simulink model "Shanthan_Heeirthan_EE469S3D_R45 (1)"  (R2023a)
settings: Solver=FixedStepDiscrete  StartTime=0.0  StopTime=120  FixedStep=dt0  RelTol=1e-3  EnableMultiTasking=on
PostLoadFcn:
  | %Set the size for the model
  | set_param(gcs,'Location',[10 10 1270 970])
  | %Set the zoom factor for the model
  | set_param(gcs,'ZoomFactor','100')
InitFcn:
  | tic
  | % Students Add call to their M-file HERE
  | Shanthan_Heeirthan_EE460_Final
  | INIT_S3D_01
StartFcn:
  | tend0=toc;
  | tic;
StopFcn:
  | tend=toc;
  | disp(['Simulation time = ' num2str(tout(end)) ' sec'])
  | disp(['Real time = ' num2str(tend) ' sec'])
  | title('DONE')
  | SCORE=round((max(0,120-tout(end)-tend0))*4+10*(40-FuelBurned)+sum(100*double(PDONE)-100*double(PDONE<.5)));
  | PlotS3D(PlotInput);
  | text(15,22,['S: ' num2str(SCORE)]);
values from neighbouring files (symbols this model uses):
  A = [0 1 0 0 0 0 ... (first row only)    [Shanthan_Heeirthan_EE460_Final (1).m]
  B = [0 0 0 ... (first row only)    [Shanthan_Heeirthan_EE460_Final (1).m]
  bm = [1 1 -1 -1 0 0 0 0; 0 0 0 0 -1 1 1 -1; -1 1 -1 1 3 -3 3 -3]    [Shanthan_Heeirthan_EE460_Final (1).m]
  C = [1 0 0 0 0 0 ... (first row only)    [Shanthan_Heeirthan_EE460_Final (1).m]
  D = [0 0 0 ... (first row only)    [Shanthan_Heeirthan_EE460_Final (1).m]
  Denchptheta = TFchptheta.Den{1}    [Shanthan_Heeirthan_EE460_Final (1).m]
  Denchpxy = TFchpxy.Den{1}    [Shanthan_Heeirthan_EE460_Final (1).m]
  Denclptheta = TFclptheta.Den{1}    [Shanthan_Heeirthan_EE460_Final (1).m]
  Denclpxy = TFclpxy.Den{1}    [Shanthan_Heeirthan_EE460_Final (1).m]
  Denlp = TFlp.Den{1}    [Shanthan_Heeirthan_EE460_Final (1).m]
  Kd = 2.1+0    (= 2.1)    [Shanthan_Heeirthan_EE460_Final (1).m]
  Ki = 0.0001    [Shanthan_Heeirthan_EE460_Final (1).m]
  Kp = 1.1+0.2    (= 1.3)    [Shanthan_Heeirthan_EE460_Final (1).m]
  L = place(A',C',ep)'    [Shanthan_Heeirthan_EE460_Final (1).m]
  Numchptheta = TFchptheta.Num{1}    [Shanthan_Heeirthan_EE460_Final (1).m]
  Numchpxy = TFchpxy.Num{1}    [Shanthan_Heeirthan_EE460_Final (1).m]
  Numclptheta = TFclptheta.Num{1}    [Shanthan_Heeirthan_EE460_Final (1).m]
  Numclpxy = TFclpxy.Num{1}    [Shanthan_Heeirthan_EE460_Final (1).m]
  Numlp = TFlp.Num{1}    [Shanthan_Heeirthan_EE460_Final (1).m]
  Pnewdata = [LVL.P1 LVL.P2 LVL.P3 LVL.P4]    [Shanthan_Heeirthan_EE460_Final (1).m]
  Sconfig = 1    [Shanthan_Heeirthan_EE460_Final (1).m]
  TFP1 = 2    [Shanthan_Heeirthan_EE460_Final (1).m]
  TFP1z = 1    [Shanthan_Heeirthan_EE460_Final (1).m]
  TFP2 = 2    [Shanthan_Heeirthan_EE460_Final (1).m]
  TFP2z = 1    [Shanthan_Heeirthan_EE460_Final (1).m]
  TFP3 = 2    [Shanthan_Heeirthan_EE460_Final (1).m]
  TFP3z = 1    [Shanthan_Heeirthan_EE460_Final (1).m]
  TFP4 = 2    [Shanthan_Heeirthan_EE460_Final (1).m]
  TFP4z = 1    [Shanthan_Heeirthan_EE460_Final (1).m]
  wcf = 2    [Shanthan_Heeirthan_EE460_Final (1).m]
  wcft = 10    [Shanthan_Heeirthan_EE460_Final (1).m]
undefined symbols (not defined in the file or in its folder): d2r, DiscIntNeverNeededParam, dt, dt0, fr, HM_S, HM_U, J, Jbase, JC0, L13, L24, LVL, M, M1, M2, M3, M4, mdti, Pdata, PTvec, r2d, SLIM, SQ, SSF, TOLdata, ULIM
libraries: simulink x85, aerolibanimutils x1, matrix_library x1
(part 1 of 7)
settings Model: Creator=bordignk  LastModifiedBy=shanthah
settings SolverCC: AlgebraicLoopSolver=TrustRegion  AutoInsertRateTranBlk=on
settings DataIOCC: LimitDataPoints=on  SaveFormat=Array  ReturnWorkspaceOutputs=off
settings OptimizationCC: LifeSpan=inf
settings DebuggingCC: CheckSSInitialOutputMsg=off  UnderspecifiedInitializationDetection=Classic  MergeDetectMultiDrivingBlocksExec=none  ParameterPrecisionLossMsg=none  AllowSymbolicDim=off  StateNameClashWarn=warning  SFUnexpectedBacktrackingDiag=warning  SFNoUnconditionalDefaultTransitionDiag=warning  SFExecutionAtInitializationDiag=none  ArithmeticOperatorsInVariantConditions=warning
settings HardwareCC: ProdBitPerPointer=32  ProdBitPerSizeT=32  ProdBitPerPtrDiffT=32  ProdLargestAtomicFloat=None  ProdIntDivRoundTo=Undefined  ProdEndianess=Unspecified  ProdWordSize=32  ProdHWDeviceType=32-bit Generic
settings ModelReferenceCC: EnableRefExpFcnMdlSchedulingChecks=on  PropagateSignalLabelsOutOfModel=off
settings SFSimCC: SimUseLocalCustomCode=off  CustomCodeUndefinedFunction=UseInterfaceOnly
settings RTWCC: RTWUseLocalCustomCode=off  DLArmComputeVersion=19.05
settings CodeAppCC: StateflowObjectComments=on
settings GRTTargetCC: TargetLangStandard=C89/C90 (ANSI)
settings ConfigComp: CovMetricSettings=dw  CovSaveCumulativeToWorkspaceVar=on  CovSaveSingleToWorkspaceVar=on  CovExternalEMLEnable=off

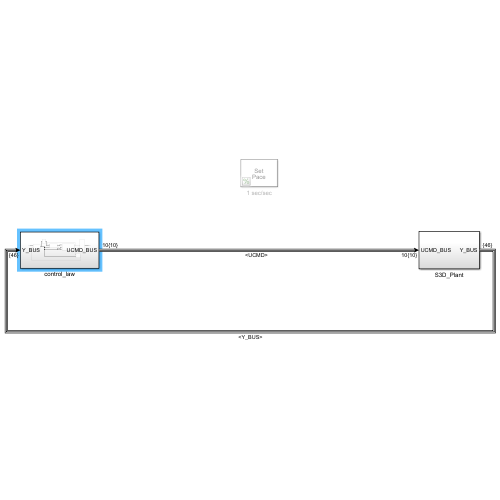
[thumbnail: Simulink's stored preview of the top-level diagram]
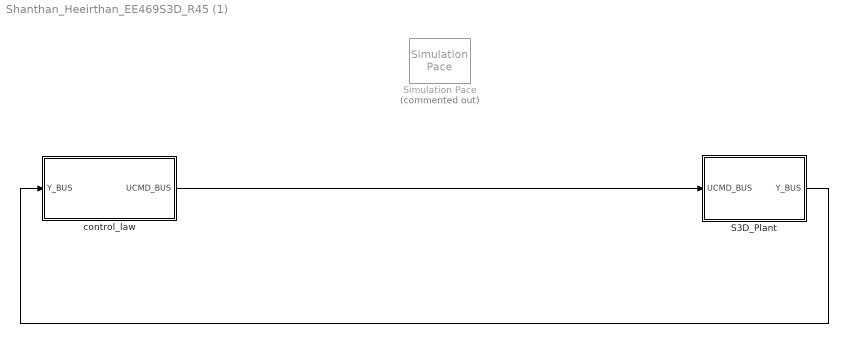
== system Shanthan_Heeirthan_EE469S3D_R45 (1) ==
  S3D_Plant : Subsystem
  Simulation Pace : aerolibanimutils/Simulation Pace  Commented=on  SimulationPace=1  SleepMode=MATLAB Thread  OutputPaceError=off  SampleTime=-1
      settings: AttributesFormatString=%<SimulationPace> sec/sec
  control_law : Subsystem
  wires:
  control_law/1(UCMD_BUS) -> S3D_Plant/1(UCMD_BUS)
  S3D_Plant/1(Y_BUS) -> control_law/1(Y_BUS)

== system Shanthan_Heeirthan_EE469S3D_R45 (1)/S3D_Plant ==
  UCMD_BUS : Inport
  Comm : Subsystem
  GetAccel : Subsystem
  Integrate : Subsystem
  MassProperties : Subsystem
  OutputDataProcessing : Subsystem
  Sensors : Subsystem
  ThrusterValues : Subsystem
  Y_BUS : Outport
  wires:
  Integrate/1(XCentroid) -> OutputDataProcessing/4(x), Comm/1(X), Sensors/1(X), GetAccel/3(X)
  MassProperties/1(MP) -> OutputDataProcessing/1(MP), Integrate/1(MP), GetAccel/1(MP), ThrusterValues/1(MP)
  OutputDataProcessing/1(Y_BUS) -> Y_BUS/1
  Comm/1(COMM) -> OutputDataProcessing/3(COMM)
  Sensors/1(Sensors) -> OutputDataProcessing/2(Sensors)
  ThrusterValues/1(U) -> MassProperties/1(U), OutputDataProcessing/5(U), GetAccel/2(U)
  GetAccel/1(ACCEL) -> Integrate/2(ACCEL)
  UCMD_BUS/1 -> ThrusterValues/2(UCMD_BUS)

== system Shanthan_Heeirthan_EE469S3D_R45 (1)/control_law ==
  Y_BUS : Inport
  Bus Selector : BusSelector  OutputSignals=Ufail  OutputAsBus=on
  CMD : Subsystem
  InputDataConditioning : Subsystem
  Observer : Subsystem
  OutputDataConditioning : Subsystem
  Regulator : Subsystem
  thrustercmd : Subsystem
  UCMD_BUS : Outport
  wires:
  Y_BUS/1 -> InputDataConditioning/1(Y_BUS)
  OutputDataConditioning/1(UCMD_BUS) -> UCMD_BUS/1
  thrustercmd/1(U_lim) -> Regulator/1(U_lim), OutputDataConditioning/1(U_lim)
  InputDataConditioning/1(Y_IN) -> Observer/2(Y_IN), Bus Selector/1, thrustercmd/3(Y_IN), Regulator/3(Y_IN), CMD/1(Y_IN)
  Regulator/1(Up) -> thrustercmd/1(Up)
  CMD/1(CMD) -> Regulator/2(CMD)
  thrustercmd/2(CAout) -> Observer/1(CAout)
  Observer/1(xhat) -> InputDataConditioning/2(x_hat)
  Bus Selector/1 -> thrustercmd/2(Ufail)  "Ufail"

== system Shanthan_Heeirthan_EE469S3D_R45 (1)/S3D_Plant/Comm ==
  X : Inport
  Bus Creator : BusCreator  Inputs=8
  Bus Selector : BusSelector  OutputSignals=P1Done,P2Done,P3Done,P4Done  OutputAsBus=on
  Bus Selector1 : BusSelector  OutputSignals=P1Done,P2Done,P3Done,P4Done  OutputAsBus=on
  Compare To Constant : simulink/Logic and Bit Operations/Compare To Constant  relop=>=  const=4  OutDataTypeStr=boolean
  Data Type Conversion : DataTypeConversion  OutDataTypeStr=uint8  SaturateOnIntegerOverflow=off  RndMeth=Floor
  P1 : Subsystem  mask{Pdx=1}
      mask prompts: Pdx "Data Point (1-4)"
  P2 : Subsystem  mask{Pdx=2}
      mask prompts: Pdx "Data Point (1-4)"
  P3 : Subsystem  mask{Pdx=3}
      mask prompts: Pdx "Data Point (1-4)"
  P4 : Subsystem  mask{Pdx=4}
      mask prompts: Pdx "Data Point (1-4)"
  Stop Simulation : Stop
  Sum of Elements : Sum  Inputs=+
  To Workspace : ToWorkspace  VariableName=PDONE  SampleTime=dt0
      settings: MaxDataPoints=1
  COMM : Outport
  wires:
  Compare To Constant/1 -> Stop Simulation/1
  Sum of Elements/1 -> Compare To Constant/1
  Data Type Conversion/1 -> Sum of Elements/1
  Bus Selector1/1 -> Data Type Conversion/1
  Bus Selector/1 -> To Workspace/1  "PDONE"
  Bus Creator/1 -> COMM/1, Bus Selector/1, Bus Selector1/1  "COMM"
  P4/1(COMM_OK) -> Bus Creator/7  "P4OK"
  P4/2(COMM_DONE) -> Bus Creator/8  "P4Done"
  P3/1(COMM_OK) -> Bus Creator/5  "P3OK"
  P3/2(COMM_DONE) -> Bus Creator/6  "P3Done"
  P2/1(COMM_OK) -> Bus Creator/3  "P2OK"
  P2/2(COMM_DONE) -> Bus Creator/4  "P2Done"
  P1/2(COMM_DONE) -> Bus Creator/2  "P1Done"
  P1/1(COMM_OK) -> Bus Creator/1  "P1OK"
  X/1 -> P3/1(X), P4/1(X), P2/1(X), P1/1(X)

== system Shanthan_Heeirthan_EE469S3D_R45 (1)/S3D_Plant/GetAccel ==
  MP : Inport
  U : Inport  Port=2
  X : Inport  Port=3
  Bus Creator : BusCreator  Inputs=3
  GetFxb : Subsystem
  GetFyb : Subsystem
  GetMz : Subsystem
  InertialAccel : Subsystem
  ACCEL : Outport
  wires:
  InertialAccel/1(ACCEL) -> ACCEL/1
  Bus Creator/1 -> InertialAccel/1(FM)  "FM"
  MP/1 -> GetMz/2(MP), InertialAccel/2(MP)
  X/1 -> InertialAccel/3(X)
  U/1 -> GetFxb/1(U), GetFyb/1(U), GetMz/1(U)
  GetFxb/1(Fxb) -> Bus Creator/1
  GetFyb/1(Fyb) -> Bus Creator/2
  GetMz/1(Mzb) -> Bus Creator/3

== system Shanthan_Heeirthan_EE469S3D_R45 (1)/S3D_Plant/Integrate ==
  MP : Inport
  ACCEL : Inport  Port=2
  ABM_INT1 : Subsystem
  Bus Creator : BusCreator  Inputs=9
  Bus Selector2 : BusSelector  OutputSignals=xddt_mps2,yddt_mps2,thtddt_rps2
  Bus to Vector1 : BusToVector
  CentroidData : Subsystem
  Demux : Demux  Outputs=6
  Mux : Mux  Inputs=2
  Selector : Selector  InputPortWidth=6  IndexOptions=Index vector (dialog)  Indices=[4 5 6]  OutputSizes=1
  XCentroid : Outport
  wires:
  CentroidData/1(XCentroid) -> XCentroid/1
  MP/1 -> CentroidData/1(MP)
  Bus Selector2/3 -> Bus Creator/9  "<thtddt_rps2>"
  Bus Selector2/1 -> Bus Creator/7  "<xddt_mps2>"
  Bus Selector2/2 -> Bus Creator/8  "<yddt_mps2>"
  Bus to Vector1/1 -> Mux/2
  Bus Creator/1 -> CentroidData/2(XCG)  "XCG"
  Selector/1 -> Mux/1
  ACCEL/1 -> Bus to Vector1/1, Bus Selector2/1
  Demux/4 -> Bus Creator/4  "xdt_mps"
  Demux/6 -> Bus Creator/6  "thtdt_rps"
  Demux/5 -> Bus Creator/5  "ydt_mps"
  Demux/2 -> Bus Creator/2  "y_m"
  Demux/1 -> Bus Creator/1  "x_m"
  Demux/3 -> Bus Creator/3  "tht_rad"
  Mux/1 -> ABM_INT1/1(DX)  "DX"
  ABM_INT1/1(X) -> Selector/1, Demux/1

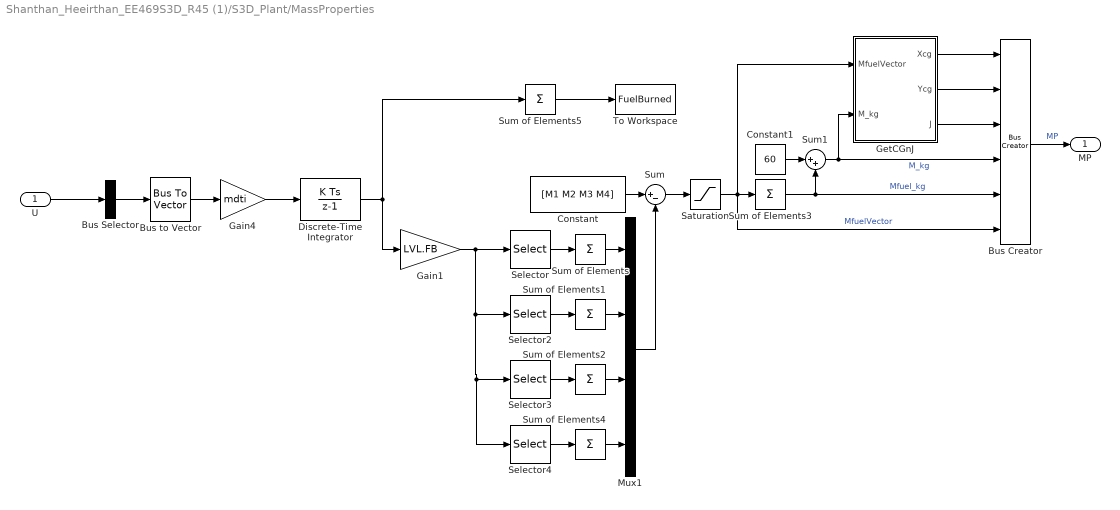
== system Shanthan_Heeirthan_EE469S3D_R45 (1)/S3D_Plant/MassProperties ==
  U : Inport
  Bus Creator : BusCreator  Inputs=6
  Bus Selector : BusSelector  OutputSignals=U1,U2,U3,U4,U5,U6,U7,U8  OutputAsBus=on
  Bus to Vector : BusToVector
  Constant : Constant  Value=[M1 M2 M3 M4]  SampleTime=dt0
  Constant1 : Constant  Value=60  SampleTime=dt0
  Discrete-Time Integrator : DiscreteIntegrator  SampleTime=dt0  UpperSaturationLimit=10  LowerSaturationLimit=0  ICPrevOutput=DiscIntNeverNeededParam  ICPrevScaledInput=DiscIntNeverNeededParam
  Gain1 : Gain  Gain=LVL.FB
  Gain4 : Gain  Gain=mdti
  GetCGnJ : Subsystem
  Mux1 : Mux
  Saturation : Saturate  UpperLimit=10  LowerLimit=0
  Selector : Selector  InputPortWidth=8  IndexOptions=Index vector (dialog)  Indices=[1 5]  OutputSizes=1
  Selector2 : Selector  InputPortWidth=8  IndexOptions=Index vector (dialog)  Indices=[2 6]  OutputSizes=1
  Selector3 : Selector  InputPortWidth=8  IndexOptions=Index vector (dialog)  Indices=[3 7]  OutputSizes=1
  Selector4 : Selector  InputPortWidth=8  IndexOptions=Index vector (dialog)  Indices=[4 8]  OutputSizes=1
  Sum : Sum  Inputs=|+-
  Sum of Elements{,1..5} (6 alike) : Sum  Inputs=+
  Sum1 : Sum  Inputs=|++
  To Workspace : ToWorkspace  VariableName=FuelBurned  SampleTime=dt0
      settings: MaxDataPoints=1
  MP : Outport
  wires:
  Gain1/1 -> Selector/1, Selector2/1, Selector3/1, Selector4/1
  Bus Creator/1 -> MP/1  "MP"
  GetCGnJ/3(J) -> Bus Creator/3
  GetCGnJ/2(Ycg) -> Bus Creator/2
  GetCGnJ/1(Xcg) -> Bus Creator/1
  Sum1/1 -> GetCGnJ/2(M_kg), Bus Creator/4  "M_kg"
  Sum of Elements3/1 -> Bus Creator/5, Sum1/2  "Mfuel_kg"
  Constant1/1 -> Sum1/1
  Saturation/1 -> Sum of Elements3/1, GetCGnJ/1(MfuelVector), Bus Creator/6  "MfuelVector"
  Sum/1 -> Saturation/1
  Constant/1 -> Sum/1
  Bus Selector/1 -> Bus to Vector/1
  U/1 -> Bus Selector/1
  Sum of Elements/1 -> Mux1/1
  Selector4/1 -> Sum of Elements4/1
  Selector3/1 -> Sum of Elements2/1
  Sum of Elements1/1 -> Mux1/2
  Sum of Elements2/1 -> Mux1/3
  Sum of Elements4/1 -> Mux1/4
  Mux1/1 -> Sum/2
  Gain4/1 -> Discrete-Time Integrator/1
  Selector/1 -> Sum of Elements/1
  Selector2/1 -> Sum of Elements1/1
  Bus to Vector/1 -> Gain4/1
  Discrete-Time Integrator/1 -> Sum of Elements5/1, Gain1/1
  Sum of Elements5/1 -> To Workspace/1

== system Shanthan_Heeirthan_EE469S3D_R45 (1)/S3D_Plant/OutputDataProcessing ==
  MP : Inport
  Sensors : Inport  Port=2
  COMM : Inport  Port=3
  x : Inport  Port=4
  U : Inport  Port=5
  Bus Creator1 : BusCreator  Inputs=46
  Bus Selector : BusSelector  OutputSignals=U1,U2,U3,U4,U5,U6,U7,U8,U9,U10,U1fail,U2fail,U3fail,U4fail,U5fail,U6fail,U7fail,U8fail,U9fail,U10fail
  Bus Selector1 : BusSelector  OutputSignals=Sensor1,Sensor2,Sensor3,Sensor4,Sensor5,Sensor6,Sensor7,Sensor8,Sensor9,S1fail,S2fail,S3fail,S4fail,S5fail,S6fail,S7fail,S8fail,S9fail
  Bus Selector2 : BusSelector  OutputSignals=P1OK,P1Done,P2OK,P2Done,P3OK,P3Done,P4OK,P4Done
  Data Type Conversion{,1..9} (10 alike) : DataTypeConversion  OutDataTypeStr=uint8  SaturateOnIntegerOverflow=off  RndMeth=Floor
  MakePlot : Subsystem
  Rate Transition : RateTransition  OutPortSampleTime=dt
  Unit Delay : UnitDelay  SampleTime=dt0  HasFrameUpgradeWarning=on
  Y_BUS : Outport
  wires:
  x/1 -> MakePlot/4(x)
  MP/1 -> MakePlot/3(MP)
  Data Type Conversion9/1 -> Bus Creator1/28  "U10est"
  Data Type Conversion8/1 -> Bus Creator1/27  "U9est"
  Data Type Conversion7/1 -> Bus Creator1/26  "U8est"
  Data Type Conversion6/1 -> Bus Creator1/25  "U7est"
  Data Type Conversion5/1 -> Bus Creator1/24  "U6est"
  Data Type Conversion4/1 -> Bus Creator1/23  "U5est"
  Data Type Conversion3/1 -> Bus Creator1/22  "U4est"
  Data Type Conversion2/1 -> Bus Creator1/21  "U3est"
  Data Type Conversion1/1 -> Bus Creator1/20  "U2est"
  Data Type Conversion/1 -> Bus Creator1/19  "U1est"
  Bus Selector1/16 -> Bus Creator1/16  "<S7fail>"
  Bus Selector1/18 -> Bus Creator1/18  "<S9fail>"
  Bus Selector1/15 -> Bus Creator1/15  "<S6fail>"
  Bus Selector1/14 -> Bus Creator1/14  "<S5fail>"
  Bus Selector1/13 -> Bus Creator1/13  "<S4fail>"
  Bus Selector1/12 -> Bus Creator1/12  "<S3fail>"
  Bus Selector1/11 -> Bus Creator1/11  "<S2fail>"
  Bus Selector1/10 -> Bus Creator1/10  "<S1fail>"
  Bus Selector1/9 -> Bus Creator1/9  "<Sensor9>"
  Bus Selector1/8 -> Bus Creator1/8  "<Sensor8>"
  Bus Selector1/6 -> Bus Creator1/6  "<Sensor6>"
  Bus Selector1/1 -> Bus Creator1/1  "<Sensor1>"
  Bus Selector1/2 -> Bus Creator1/2  "<Sensor2>"
  Bus Selector1/17 -> Bus Creator1/17  "<S8fail>"
  Bus Selector1/3 -> Bus Creator1/3  "<Sensor3>"
  Bus Selector1/4 -> Bus Creator1/4  "<Sensor4>"
  Bus Selector1/5 -> Bus Creator1/5  "<Sensor5>"
  Bus Selector1/7 -> Bus Creator1/7  "<Sensor7>"
  Bus Selector/11 -> Bus Creator1/29  "<U1fail>"
  Bus Selector/16 -> Bus Creator1/34  "<U6fail>"
  Bus Selector/13 -> Bus Creator1/31  "<U3fail>"
  Bus Selector/15 -> Bus Creator1/33  "<U5fail>"
  Bus Selector/20 -> Bus Creator1/38  "<U10fail>"
  Bus Selector/1 -> Data Type Conversion/1  "<U1>"
  Bus Selector/18 -> Bus Creator1/36  "<U8fail>"
  Bus Selector/2 -> Data Type Conversion1/1  "<U2>"
  Bus Selector/19 -> Bus Creator1/37  "<U9fail>"
  Bus Selector/12 -> Bus Creator1/30  "<U2fail>"
  Bus Selector/4 -> Data Type Conversion3/1  "<U4>"
  Bus Selector/17 -> Bus Creator1/35  "<U7fail>"
  Bus Selector/14 -> Bus Creator1/32  "<U4fail>"
  Bus Selector/10 -> Data Type Conversion9/1  "<U10>"
  Bus Selector/8 -> Data Type Conversion7/1  "<U8>"
  Bus Selector/9 -> Data Type Conversion8/1  "<U9>"
  Bus Selector/7 -> Data Type Conversion6/1  "<U7>"
  Bus Selector/6 -> Data Type Conversion5/1  "<U6>"
  Bus Selector/5 -> Data Type Conversion4/1  "<U5>"
  Bus Selector/3 -> Data Type Conversion2/1  "<U3>"
  Rate Transition/1 -> Y_BUS/1  "Y_BUS"
  Unit Delay/1 -> Rate Transition/1
  Bus Selector2/7 -> Bus Creator1/45  "<P4OK>"
  Bus Selector2/4 -> Bus Creator1/42  "<P2Done>"
  Bus Selector2/6 -> Bus Creator1/44  "<P3Done>"
  Bus Selector2/1 -> Bus Creator1/39  "<P1OK>"
  Bus Selector2/2 -> Bus Creator1/40  "<P1Done>"
  Bus Selector2/5 -> Bus Creator1/43  "<P3OK>"
  Bus Selector2/3 -> Bus Creator1/41  "<P2OK>"
  Bus Selector2/8 -> Bus Creator1/46  "<P4Done>"
  COMM/1 -> Bus Selector2/1, MakePlot/5(COMM)
  Sensors/1 -> MakePlot/2(Sensors), Bus Selector1/1
  U/1 -> Bus Selector/1, MakePlot/1(U)
  Bus Creator1/1 -> Unit Delay/1

== system Shanthan_Heeirthan_EE469S3D_R45 (1)/S3D_Plant/Sensors ==
  X : Inport
  CASE1 : Subsystem  TreatAsAtomicUnit=on
  CASE2 : Subsystem  TreatAsAtomicUnit=on
  CASE3 : Subsystem  TreatAsAtomicUnit=on
  Constant : Constant  Value=Sconfig  SampleTime=dt0
  ConvertINT16 : Subsystem
  HealthMonitoring : Subsystem
  Merge : Merge  Inputs=3
  Switch Case : SwitchCase  CaseConditions={1,2}  SampleTime=dt0
  Sensors : Outport
  wires:
  HealthMonitoring/1(Sensors) -> Sensors/1
  ConvertINT16/1(INT16) -> HealthMonitoring/1(SensorValues)
  Merge/1 -> ConvertINT16/1(SDouble)  "SDouble"
  X/1 -> CASE1/1(X), CASE2/1(X), CASE3/1(X)
  CASE3/1(Out1) -> Merge/3
  CASE2/1(Out1) -> Merge/2
  CASE1/1(Out1) -> Merge/1
  Switch Case/3 -> CASE3/Action
  Switch Case/2 -> CASE2/Action
  Switch Case/1 -> CASE1/Action
  Constant/1 -> Switch Case/1

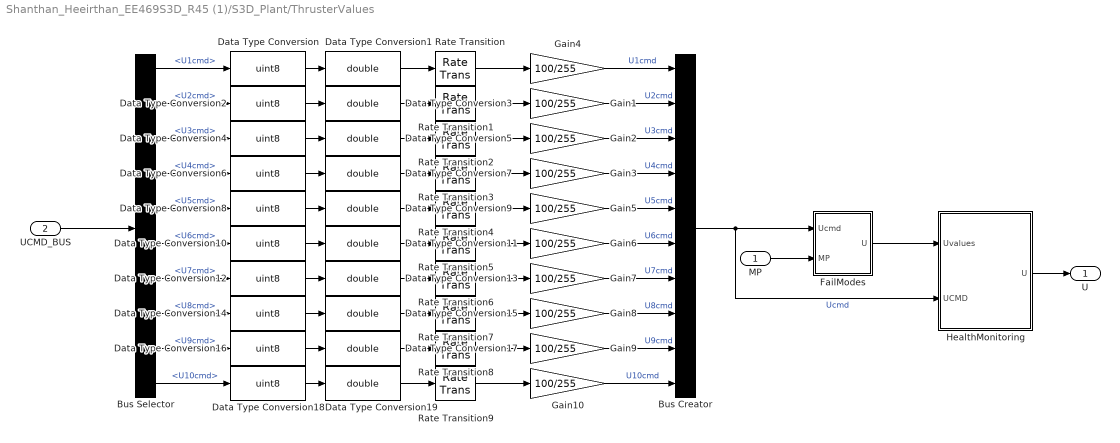
== system Shanthan_Heeirthan_EE469S3D_R45 (1)/S3D_Plant/ThrusterValues ==
  MP : Inport
  UCMD_BUS : Inport  Port=2
  Bus Creator : BusCreator  Inputs=10
  Bus Selector : BusSelector  OutputSignals=U1cmd,U2cmd,U3cmd,U4cmd,U5cmd,U6cmd,U7cmd,U8cmd,U9cmd,U10cmd
  Data Type Conversion{,2,4,6,8,10,12,14,16,18} (10 alike) : DataTypeConversion  OutDataTypeStr=uint8  SaturateOnIntegerOverflow=off  RndMeth=Floor
  Data Type Conversion{1,3,5,7,9,11,13,15,17,19} (10 alike) : DataTypeConversion  OutDataTypeStr=double  SaturateOnIntegerOverflow=off  RndMeth=Floor
  FailModes : Subsystem
  Gain{1..10} (10 alike) : Gain  Gain=100/255
  HealthMonitoring : Subsystem
  Rate Transition{,1..9} (10 alike) : RateTransition  OutPortSampleTime=dt0
  U : Outport
  wires:
  Rate Transition9/1 -> Gain10/1
  Rate Transition8/1 -> Gain9/1
  Rate Transition7/1 -> Gain8/1
  Rate Transition6/1 -> Gain7/1
  Rate Transition5/1 -> Gain6/1
  Rate Transition4/1 -> Gain5/1
  Rate Transition3/1 -> Gain3/1
  Rate Transition2/1 -> Gain2/1
  Rate Transition1/1 -> Gain1/1
  Rate Transition/1 -> Gain4/1
  HealthMonitoring/1(U) -> U/1
  FailModes/1(U) -> HealthMonitoring/1(Uvalues)
  MP/1 -> FailModes/2(MP)
  Gain10/1 -> Bus Creator/10  "U10cmd"
  Gain9/1 -> Bus Creator/9  "U9cmd"
  Bus Selector/10 -> Data Type Conversion18/1  "<U10cmd>"
  Bus Selector/9 -> Data Type Conversion16/1  "<U9cmd>"
  Data Type Conversion19/1 -> Rate Transition9/1
  Data Type Conversion18/1 -> Data Type Conversion19/1
  Data Type Conversion17/1 -> Rate Transition8/1
  Data Type Conversion16/1 -> Data Type Conversion17/1
  Bus Creator/1 -> FailModes/1(Ucmd), HealthMonitoring/2(UCMD)  "Ucmd"
  Gain8/1 -> Bus Creator/8  "U8cmd"
  Gain7/1 -> Bus Creator/7  "U7cmd"
  Gain6/1 -> Bus Creator/6  "U6cmd"
  Gain5/1 -> Bus Creator/5  "U5cmd"
  Gain3/1 -> Bus Creator/4  "U4cmd"
  Gain2/1 -> Bus Creator/3  "U3cmd"
  Gain1/1 -> Bus Creator/2  "U2cmd"
  Gain4/1 -> Bus Creator/1  "U1cmd"
  Bus Selector/8 -> Data Type Conversion14/1  "<U8cmd>"
  Bus Selector/7 -> Data Type Conversion12/1  "<U7cmd>"
  Bus Selector/6 -> Data Type Conversion10/1  "<U6cmd>"
  Bus Selector/5 -> Data Type Conversion8/1  "<U5cmd>"
  Bus Selector/4 -> Data Type Conversion6/1  "<U4cmd>"
  Bus Selector/3 -> Data Type Conversion4/1  "<U3cmd>"
  Data Type Conversion15/1 -> Rate Transition7/1
  Data Type Conversion14/1 -> Data Type Conversion15/1
  Data Type Conversion13/1 -> Rate Transition6/1
  Data Type Conversion12/1 -> Data Type Conversion13/1
  Data Type Conversion11/1 -> Rate Transition5/1
  Data Type Conversion10/1 -> Data Type Conversion11/1
  Data Type Conversion9/1 -> Rate Transition4/1
  Data Type Conversion8/1 -> Data Type Conversion9/1
  Data Type Conversion7/1 -> Rate Transition3/1
  Data Type Conversion6/1 -> Data Type Conversion7/1
  Data Type Conversion5/1 -> Rate Transition2/1
  Data Type Conversion4/1 -> Data Type Conversion5/1
  Bus Selector/2 -> Data Type Conversion2/1  "<U2cmd>"
  Data Type Conversion3/1 -> Rate Transition1/1
  Data Type Conversion2/1 -> Data Type Conversion3/1
  Data Type Conversion1/1 -> Rate Transition/1
  Data Type Conversion/1 -> Data Type Conversion1/1
  Bus Selector/1 -> Data Type Conversion/1  "<U1cmd>"
  UCMD_BUS/1 -> Bus Selector/1

== system Shanthan_Heeirthan_EE469S3D_R45 (1)/control_law/CMD ==
  Y_IN : Inport
  CMDprocess : Subsystem
  CMD : Outport
  wires:
  Y_IN/1 -> CMDprocess/1(Y_IN)
  CMDprocess/1(CMD) -> CMD/1

== system Shanthan_Heeirthan_EE469S3D_R45 (1)/control_law/InputDataConditioning ==
  Y_BUS : Inport
  x_hat : Inport  Port=2
  Bus Creator2 : BusCreator  Inputs=4
  Bus Selector : BusSelector  OutputSignals=U1fail,U2fail,U3fail,U4fail,U5fail,U6fail,U7fail,U8fail  OutputAsBus=on
  Bus Selector1 : BusSelector  OutputSignals=P1Done,P2Done,P3Done,P4Done  OutputAsBus=on
  Bus Selector2 : BusSelector  OutputSignals=S1fail,S2fail,S3fail,S4fail,S5fail,S6fail,S7fail,S8fail,S9fail,Sensor1,Sensor2,Sensor3,Sensor4,Sensor5,Sensor6,Sensor7,Sensor8,Sensor9  OutputAsBus=on
  SensorConditioning : Subsystem
  xhatsel : Subsystem
  Y_IN : Outport
  wires:
  Y_BUS/1 -> Bus Selector/1, Bus Selector2/1, Bus Selector1/1
  Bus Creator2/1 -> Y_IN/1  "Y_IN"
  x_hat/1 -> xhatsel/1(xhat)
  xhatsel/1(x_hat) -> Bus Creator2/3
  Bus Selector1/1 -> Bus Creator2/1  "Pstatus"
  SensorConditioning/1(Y_sens) -> Bus Creator2/2  "Y_IN_sens"
  Bus Selector/1 -> Bus Creator2/4  "Ufail"
  Bus Selector2/1 -> SensorConditioning/1(Y_BUS)  "Y_BUS"

== system Shanthan_Heeirthan_EE469S3D_R45 (1)/control_law/Observer ==
  CAout : Inport
  Y_IN : Inport  Port=2
  Bus Selector : BusSelector  OutputSignals=Y_IN_sens.X1_m,Y_IN_sens.theta_degps2,Y_IN_sens.X_mps,Y_IN_sens.X_mps2,Y_IN_sens.Y_m,Y_IN_sens.Y_mps,Y_IN_sens.Y_mps2,Y_IN_sens.theta_deg,Y_IN_sens.theta_degps  OutputAsBus=on
  Bus to Vector : BusToVector
  Discrete-Time Integrator : DiscreteIntegrator  SampleTime=dt  ICPrevOutput=DiscIntNeverNeededParam  ICPrevScaledInput=DiscIntNeverNeededParam
  Gain : Gain  Gain=D  Multiplication=Matrix(K*u)
  Gain1 : Gain  Gain=B  Multiplication=Matrix(K*u)
  Gain2 : Gain  Gain=A  Multiplication=Matrix(K*u)
  Gain3 : Gain  Gain=L  Multiplication=Matrix(K*u)
  Gain4 : Gain  Gain=C  Multiplication=Matrix(K*u)
  Gain5 : Gain  Gain=[1;1;1;1;1;1;180/pi;180/pi;180/pi]
  Sum : Sum  Inputs=|++
  Sum1 : Sum  Inputs=|++
  Sum2 : Sum  Inputs=|++
  Sum3 : Sum  Inputs=-+|
  xhat : Outport
  wires:
  CAout/1 -> Gain1/1, Gain/1
  Sum1/1 -> Sum/2
  Gain3/1 -> Sum1/1
  Gain1/1 -> Sum/1
  Gain/1 -> Sum2/1
  Gain2/1 -> Sum1/2
  Sum/1 -> Discrete-Time Integrator/1  "xhat_dot"
  Discrete-Time Integrator/1 -> Gain4/1, xhat/1, Gain2/1  "xhat"
  Gain4/1 -> Sum2/2
  Sum3/1 -> Gain3/1
  Bus to Vector/1 -> Sum3/2  "Y_IN"
  Y_IN/1 -> Bus Selector/1
  Bus Selector/1 -> Bus to Vector/1  "Y_IN"
  Sum2/1 -> Gain5/1
  Gain5/1 -> Sum3/1

== system Shanthan_Heeirthan_EE469S3D_R45 (1)/control_law/OutputDataConditioning ==
  U_lim : Inport
  Bus Creator : BusCreator  Inputs=10
  Data Type Conversion{1..10} (10 alike) : DataTypeConversion  OutDataTypeStr=uint8  SaturateOnIntegerOverflow=off  RndMeth=Floor
  Demux : Demux  Outputs=10
  Gain{1..10} (10 alike) : Gain  Gain=2.55
  UCMD_BUS : Outport
  wires:
  Data Type Conversion1/1 -> Bus Creator/1  "U1cmd"
  Demux/1 -> Gain1/1  "U1cmd"
  Bus Creator/1 -> UCMD_BUS/1  "UCMD"
  Gain1/1 -> Data Type Conversion1/1
  Demux/2 -> Gain2/1  "U2cmd"
  Gain2/1 -> Data Type Conversion2/1
  Data Type Conversion2/1 -> Bus Creator/2  "U2cmd"
  Demux/4 -> Gain3/1  "U4cmd"
  Gain3/1 -> Data Type Conversion3/1
  Data Type Conversion3/1 -> Bus Creator/4  "U4cmd"
  Demux/3 -> Gain4/1  "U3cmd"
  Gain4/1 -> Data Type Conversion4/1
  Data Type Conversion4/1 -> Bus Creator/3  "U3cmd"
  Demux/6 -> Gain5/1  "U6cmd"
  Gain5/1 -> Data Type Conversion5/1
  Data Type Conversion5/1 -> Bus Creator/6  "U6cmd"
  Gain7/1 -> Data Type Conversion7/1
  Data Type Conversion7/1 -> Bus Creator/8  "U8cmd"
  Data Type Conversion9/1 -> Bus Creator/5  "U5cmd"
  Demux/5 -> Gain9/1  "U5cmd"
  Gain9/1 -> Data Type Conversion9/1
  Demux/9 -> Gain8/1  "U9cmd"
  Gain8/1 -> Data Type Conversion8/1
  Data Type Conversion8/1 -> Bus Creator/9  "U9cmd"
  Demux/10 -> Gain10/1  "U10cmd"
  Gain10/1 -> Data Type Conversion10/1
  Data Type Conversion10/1 -> Bus Creator/10  "U10cmd"
  Gain6/1 -> Data Type Conversion6/1
  Data Type Conversion6/1 -> Bus Creator/7  "U7cmd"
  Demux/7 -> Gain6/1  "U7cmd"
  Demux/8 -> Gain7/1  "U8cmd"
  U_lim/1 -> Demux/1

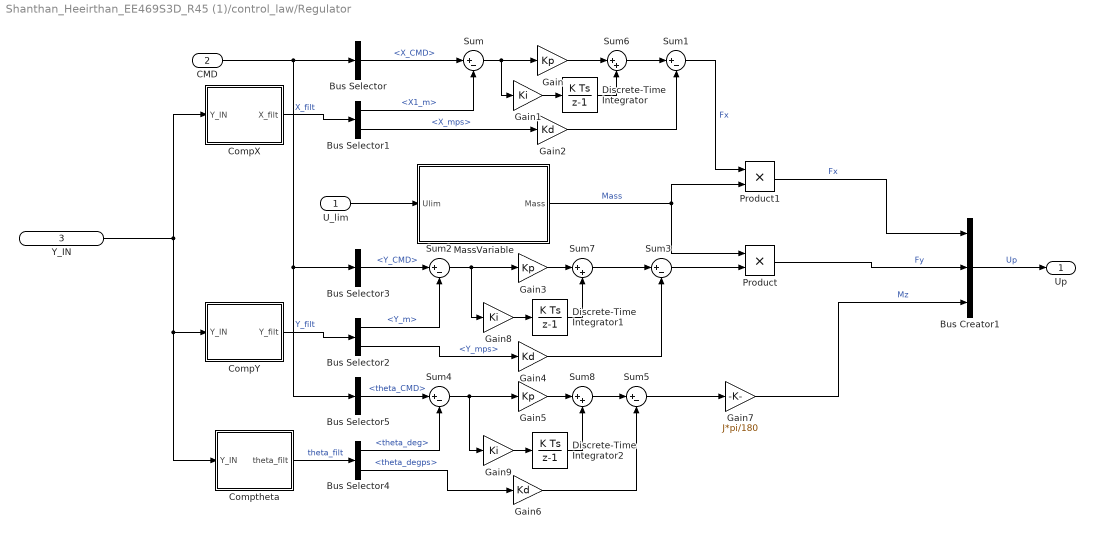
== system Shanthan_Heeirthan_EE469S3D_R45 (1)/control_law/Regulator ==
  U_lim : Inport
  CMD : Inport  Port=2
  Y_IN : Inport  Port=3
  Bus Creator1 : BusCreator  Inputs=3
  Bus Selector : BusSelector  OutputSignals=X_CMD
  Bus Selector1 : BusSelector  OutputSignals=X1_m,X_mps
  Bus Selector2 : BusSelector  OutputSignals=Y_m,Y_mps
  Bus Selector3 : BusSelector  OutputSignals=Y_CMD
  Bus Selector4 : BusSelector  OutputSignals=theta_deg,theta_degps
  Bus Selector5 : BusSelector  OutputSignals=theta_CMD
  CompX : Subsystem
  CompY : Subsystem
  Comptheta : Subsystem
  Discrete-Time Integrator : DiscreteIntegrator  SampleTime=-1  ICPrevOutput=DiscIntNeverNeededParam  ICPrevScaledInput=DiscIntNeverNeededParam
  Discrete-Time Integrator1 : DiscreteIntegrator  SampleTime=-1  ICPrevOutput=DiscIntNeverNeededParam  ICPrevScaledInput=DiscIntNeverNeededParam
  Discrete-Time Integrator2 : DiscreteIntegrator  SampleTime=-1  ICPrevOutput=DiscIntNeverNeededParam  ICPrevScaledInput=DiscIntNeverNeededParam
  Gain : Gain  Gain=Kp
  Gain1 : Gain  Gain=Ki
  Gain2 : Gain  Gain=Kd
  Gain3 : Gain  Gain=Kp
  Gain4 : Gain  Gain=Kd
  Gain5 : Gain  Gain=Kp
  Gain6 : Gain  Gain=Kd
  Gain7 : Gain  Gain=J*pi/180
  Gain8 : Gain  Gain=Ki
  Gain9 : Gain  Gain=Ki
  MassVariable : Subsystem
  Product : Product
  Product1 : Product
  Sum{,1..5} (6 alike) : Sum  Inputs=|+-
  Sum6 : Sum  Inputs=|++
  Sum7 : Sum  Inputs=|++
  Sum8 : Sum  Inputs=|++
  Up : Outport
  wires:
  CMD/1 -> Bus Selector5/1, Bus Selector3/1, Bus Selector/1
  Bus Creator1/1 -> Up/1  "Up"
  Bus Selector/1 -> Sum/1  "<X_CMD>"
  Bus Selector1/1 -> Sum/2  "<X1_m>"
  Sum/1 -> Gain/1, Gain1/1
  Bus Selector1/2 -> Gain2/1  "<X_mps>"
  Gain2/1 -> Sum1/2
  Bus Selector3/1 -> Sum2/1  "<Y_CMD>"
  Bus Selector2/1 -> Sum2/2  "<Y_m>"
  Bus Selector2/2 -> Gain4/1  "<Y_mps>"
  Gain4/1 -> Sum3/2
  Bus Selector5/1 -> Sum4/1  "<theta_CMD>"
  Bus Selector4/2 -> Gain6/1  "<theta_degps>"
  Bus Selector4/1 -> Sum4/2  "<theta_deg>"
  Gain6/1 -> Sum5/2
  Sum5/1 -> Gain7/1
  Product/1 -> Bus Creator1/2  "Fy"
  Sum3/1 -> Product/2
  MassVariable/1(Mass) -> Product1/2, Product/1  "Mass"
  Sum1/1 -> Product1/1  "Fx"
  Product1/1 -> Bus Creator1/1  "Fx"
  U_lim/1 -> MassVariable/1(Ulim)
  Gain1/1 -> Discrete-Time Integrator/1
  Discrete-Time Integrator/1 -> Sum6/2
  Gain/1 -> Sum6/1
  Sum6/1 -> Sum1/1
  Gain8/1 -> Discrete-Time Integrator1/1
  Sum2/1 -> Gain8/1, Gain3/1
  Discrete-Time Integrator1/1 -> Sum7/2
  Gain3/1 -> Sum7/1
  Sum7/1 -> Sum3/1
  Gain9/1 -> Discrete-Time Integrator2/1
  Sum4/1 -> Gain9/1, Gain5/1
  Discrete-Time Integrator2/1 -> Sum8/2
  Gain5/1 -> Sum8/1
  Sum8/1 -> Sum5/1
  Gain7/1 -> Bus Creator1/3  "Mz"
  Y_IN/1 -> CompX/1(Y_IN), Comptheta/1(Y_IN), CompY/1(Y_IN)
  Comptheta/1(theta_filt) -> Bus Selector4/1  "theta_filt"
  CompX/1(X_filt) -> Bus Selector1/1  "X_filt"
  CompY/1(Y_filt) -> Bus Selector2/1  "Y_filt"

== system Shanthan_Heeirthan_EE469S3D_R45 (1)/control_law/thrustercmd ==
  Up : Inport
  Ufail : Inport  Port=2
  Y_IN : Inport  Port=3
  Bus to Vector : BusToVector
  CAcreator : Subsystem
  Constant2 : Constant  Value=0
  DCM : Subsystem
  Demux : Demux  Outputs=8
  GenInverse : Subsystem
  Mux : Mux  Inputs=10
  Product : Product  Multiplication=Matrix(*)
  Product1 : Product  Multiplication=Matrix(*)
  Saturation8 : Saturate  UpperLimit=100  LowerLimit=0
  Transpose : Math  Operator=transpose
  U_lim : Outport
  CAout : Outport  Port=2
  wires:
  Demux/3 -> Mux/3  "U3cmd"
  Demux/2 -> Mux/2  "U2cmd"
  Demux/4 -> Mux/4  "U4cmd"
  Demux/5 -> Mux/5  "U5cmd"
  Demux/1 -> Mux/1  "U1cmd"
  Demux/6 -> Mux/6  "U6cmd"
  Mux/1 -> U_lim/1, CAcreator/2(U_lim)  "U_lim"
  Demux/7 -> Mux/7  "U7cmd"
  Demux/8 -> Mux/8  "U8cmd"
  Constant2/1 -> Mux/9, Mux/10
  Product1/1 -> Product/2  "udp"
  Saturation8/1 -> Demux/1  "tcmds"
  Product/1 -> Saturation8/1  "tcmds"
  Up/1 -> Bus to Vector/1
  CAcreator/1(CAout) -> CAout/1
  Y_IN/1 -> DCM/1(Y_IN)
  Bus to Vector/1 -> Transpose/1  "Up"
  DCM/1(IUR) -> Product1/1, CAcreator/1(DCM)  "iur"
  Transpose/1 -> Product1/2  "udp"
  GenInverse/1(ginv) -> Product/1
  Ufail/1 -> GenInverse/1(Ufail)

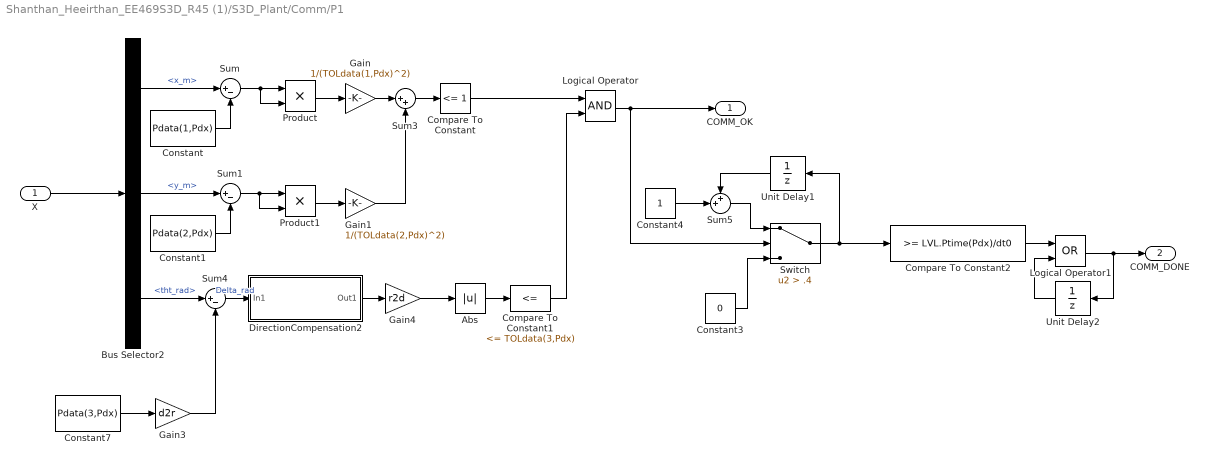
== system Shanthan_Heeirthan_EE469S3D_R45 (1)/S3D_Plant/Comm/P1 ==
  X : Inport
  Abs : Abs  SaturateOnIntegerOverflow=off
  Bus Selector2 : BusSelector  OutputSignals=x_m,y_m,tht_rad
  Compare To Constant : simulink/Logic and Bit Operations/Compare To Constant  relop=<=  const=1  OutDataTypeStr=boolean
  Compare To Constant1 : simulink/Logic and Bit Operations/Compare To Constant  relop=<=  const=TOLdata(3,Pdx)  OutDataTypeStr=boolean
  Compare To Constant2 : simulink/Logic and Bit Operations/Compare To Constant  relop=>=  const=LVL.Ptime(Pdx)/dt0  OutDataTypeStr=boolean
  Constant : Constant  Value=Pdata(1,Pdx)  SampleTime=dt0
  Constant1 : Constant  Value=Pdata(2,Pdx)  SampleTime=dt0
  Constant3 : Constant  Value=0  SampleTime=dt0
  Constant4 : Constant  SampleTime=dt0
  Constant7 : Constant  Value=Pdata(3,Pdx)  SampleTime=dt0
  DirectionCompensation2 : Subsystem
  Gain : Gain  Gain=1/(TOLdata(1,Pdx)^2)
  Gain1 : Gain  Gain=1/(TOLdata(2,Pdx)^2)
  Gain3 : Gain  Gain=d2r
  Gain4 : Gain  Gain=r2d
  Logical Operator : Logic  AllPortsSameDT=off  OutDataTypeStr=boolean
  Logical Operator1 : Logic  Operator=OR  AllPortsSameDT=off  OutDataTypeStr=boolean
  Product : Product
  Product1 : Product
  Sum : Sum  Inputs=|+-
  Sum1 : Sum  Inputs=|+-
  Sum3 : Sum  Inputs=|++
  Sum4 : Sum  Inputs=|+-
  Sum5 : Sum  Inputs=++|
  Switch : Switch  Criteria=u2 > Threshold  Threshold=.4  SaturateOnIntegerOverflow=off  InputSameDT=off
  Unit Delay1 : UnitDelay  SampleTime=dt0  HasFrameUpgradeWarning=on
  Unit Delay2 : UnitDelay  SampleTime=dt0  HasFrameUpgradeWarning=on
  COMM_OK : Outport
  COMM_DONE : Outport  Port=2
  wires:
  Gain4/1 -> Abs/1
  Sum4/1 -> DirectionCompensation2/1(In1)  "Delta_rad"
  Gain3/1 -> Sum4/2
  Constant7/1 -> Gain3/1
  Constant3/1 -> Switch/3
  Sum5/1 -> Switch/1
  Unit Delay1/1 -> Sum5/1
  Constant4/1 -> Sum5/2
  Logical Operator1/1 -> Unit Delay2/1, COMM_DONE/1
  Compare To Constant2/1 -> Logical Operator1/1
  Switch/1 -> Unit Delay1/1, Compare To Constant2/1
  Unit Delay2/1 -> Logical Operator1/2
  Sum3/1 -> Compare To Constant/1
  Compare To Constant/1 -> Logical Operator/1
  Abs/1 -> Compare To Constant1/1
  Product/1 -> Gain/1
  Compare To Constant1/1 -> Logical Operator/2
  Constant/1 -> Sum/2
  Logical Operator/1 -> Switch/2, COMM_OK/1
  Bus Selector2/1 -> Sum/1  "<x_m>"
  Bus Selector2/2 -> Sum1/1  "<y_m>"
  Constant1/1 -> Sum1/2
  X/1 -> Bus Selector2/1
  Sum1/1 -> Product1/1, Product1/2
  Gain/1 -> Sum3/1
  Sum/1 -> Product/1, Product/2
  Gain1/1 -> Sum3/2
  Bus Selector2/3 -> Sum4/1  "<tht_rad>"
  Product1/1 -> Gain1/1
  DirectionCompensation2/1(Out1) -> Gain4/1

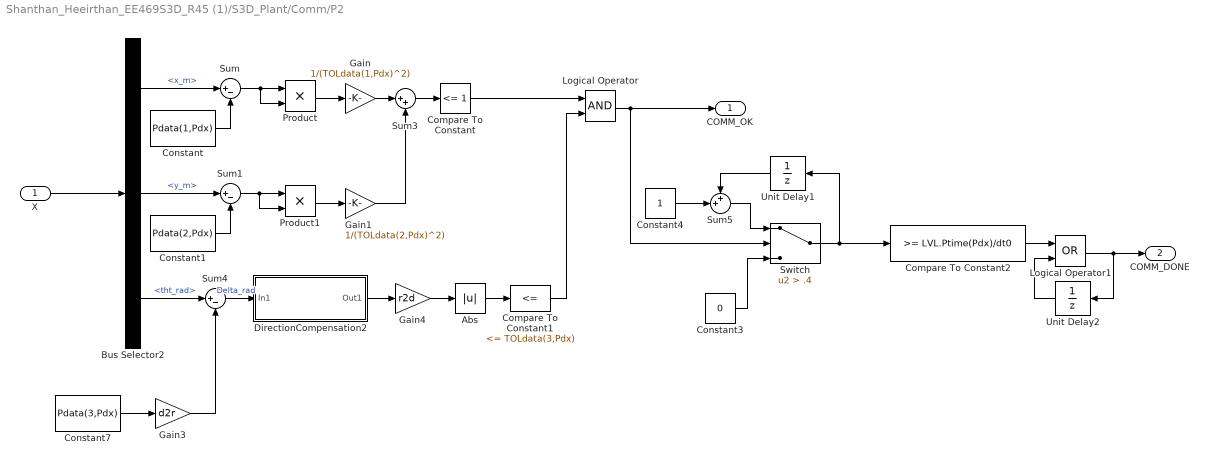
== system Shanthan_Heeirthan_EE469S3D_R45 (1)/S3D_Plant/Comm/P2 ==
  X : Inport
  Abs : Abs  SaturateOnIntegerOverflow=off
  Bus Selector2 : BusSelector  OutputSignals=x_m,y_m,tht_rad
  Compare To Constant : simulink/Logic and Bit Operations/Compare To Constant  relop=<=  const=1  OutDataTypeStr=boolean
  Compare To Constant1 : simulink/Logic and Bit Operations/Compare To Constant  relop=<=  const=TOLdata(3,Pdx)  OutDataTypeStr=boolean
  Compare To Constant2 : simulink/Logic and Bit Operations/Compare To Constant  relop=>=  const=LVL.Ptime(Pdx)/dt0  OutDataTypeStr=boolean
  Constant : Constant  Value=Pdata(1,Pdx)  SampleTime=dt0
  Constant1 : Constant  Value=Pdata(2,Pdx)  SampleTime=dt0
  Constant3 : Constant  Value=0  SampleTime=dt0
  Constant4 : Constant  SampleTime=dt0
  Constant7 : Constant  Value=Pdata(3,Pdx)  SampleTime=dt0
  DirectionCompensation2 : Subsystem
  Gain : Gain  Gain=1/(TOLdata(1,Pdx)^2)
  Gain1 : Gain  Gain=1/(TOLdata(2,Pdx)^2)
  Gain3 : Gain  Gain=d2r
  Gain4 : Gain  Gain=r2d
  Logical Operator : Logic  AllPortsSameDT=off  OutDataTypeStr=boolean
  Logical Operator1 : Logic  Operator=OR  AllPortsSameDT=off  OutDataTypeStr=boolean
  Product : Product
  Product1 : Product
  Sum : Sum  Inputs=|+-
  Sum1 : Sum  Inputs=|+-
  Sum3 : Sum  Inputs=|++
  Sum4 : Sum  Inputs=|+-
  Sum5 : Sum  Inputs=++|
  Switch : Switch  Criteria=u2 > Threshold  Threshold=.4  SaturateOnIntegerOverflow=off  InputSameDT=off
  Unit Delay1 : UnitDelay  SampleTime=dt0  HasFrameUpgradeWarning=on
  Unit Delay2 : UnitDelay  SampleTime=dt0  HasFrameUpgradeWarning=on
  COMM_OK : Outport
  COMM_DONE : Outport  Port=2
  wires:
  Gain4/1 -> Abs/1
  DirectionCompensation2/1(Out1) -> Gain4/1
  Sum4/1 -> DirectionCompensation2/1(In1)  "Delta_rad"
  Gain3/1 -> Sum4/2
  Constant7/1 -> Gain3/1
  Constant3/1 -> Switch/3
  Sum5/1 -> Switch/1
  Unit Delay1/1 -> Sum5/1
  Constant4/1 -> Sum5/2
  Logical Operator1/1 -> Unit Delay2/1, COMM_DONE/1
  Compare To Constant2/1 -> Logical Operator1/1
  Switch/1 -> Unit Delay1/1, Compare To Constant2/1
  Unit Delay2/1 -> Logical Operator1/2
  Sum3/1 -> Compare To Constant/1
  Compare To Constant/1 -> Logical Operator/1
  Abs/1 -> Compare To Constant1/1
  Product/1 -> Gain/1
  Compare To Constant1/1 -> Logical Operator/2
  Constant/1 -> Sum/2
  Logical Operator/1 -> Switch/2, COMM_OK/1
  Bus Selector2/1 -> Sum/1  "<x_m>"
  Bus Selector2/2 -> Sum1/1  "<y_m>"
  Constant1/1 -> Sum1/2
  X/1 -> Bus Selector2/1
  Sum1/1 -> Product1/1, Product1/2
  Gain/1 -> Sum3/1
  Sum/1 -> Product/1, Product/2
  Gain1/1 -> Sum3/2
  Bus Selector2/3 -> Sum4/1  "<tht_rad>"
  Product1/1 -> Gain1/1

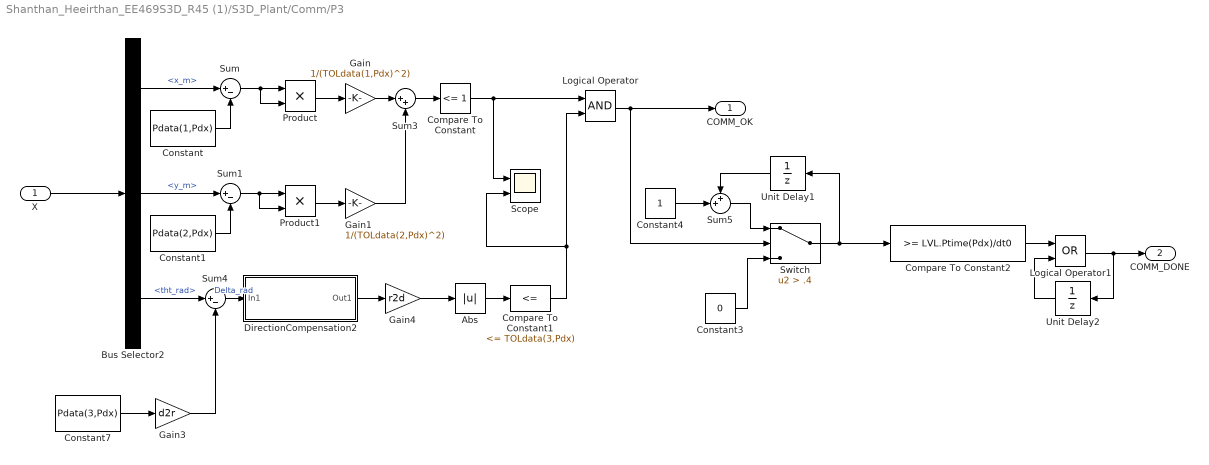
== system Shanthan_Heeirthan_EE469S3D_R45 (1)/S3D_Plant/Comm/P3 ==
  X : Inport
  Abs : Abs  SaturateOnIntegerOverflow=off
  Bus Selector2 : BusSelector  OutputSignals=x_m,y_m,tht_rad
  Compare To Constant : simulink/Logic and Bit Operations/Compare To Constant  relop=<=  const=1  OutDataTypeStr=boolean
  Compare To Constant1 : simulink/Logic and Bit Operations/Compare To Constant  relop=<=  const=TOLdata(3,Pdx)  OutDataTypeStr=boolean
  Compare To Constant2 : simulink/Logic and Bit Operations/Compare To Constant  relop=>=  const=LVL.Ptime(Pdx)/dt0  OutDataTypeStr=boolean
  Constant : Constant  Value=Pdata(1,Pdx)  SampleTime=dt0
  Constant1 : Constant  Value=Pdata(2,Pdx)  SampleTime=dt0
  Constant3 : Constant  Value=0  SampleTime=dt0
  Constant4 : Constant  SampleTime=dt0
  Constant7 : Constant  Value=Pdata(3,Pdx)  SampleTime=dt0
  DirectionCompensation2 : Subsystem
  Gain : Gain  Gain=1/(TOLdata(1,Pdx)^2)
  Gain1 : Gain  Gain=1/(TOLdata(2,Pdx)^2)
  Gain3 : Gain  Gain=d2r
  Gain4 : Gain  Gain=r2d
  Logical Operator : Logic  AllPortsSameDT=off  OutDataTypeStr=boolean
  Logical Operator1 : Logic  Operator=OR  AllPortsSameDT=off  OutDataTypeStr=boolean
  Product : Product
  Product1 : Product
  Scope : Scope  NumInputPorts=2
  Sum : Sum  Inputs=|+-
  Sum1 : Sum  Inputs=|+-
  Sum3 : Sum  Inputs=|++
  Sum4 : Sum  Inputs=|+-
  Sum5 : Sum  Inputs=++|
  Switch : Switch  Criteria=u2 > Threshold  Threshold=.4  SaturateOnIntegerOverflow=off  InputSameDT=off
  Unit Delay1 : UnitDelay  SampleTime=dt0  HasFrameUpgradeWarning=on
  Unit Delay2 : UnitDelay  SampleTime=dt0  HasFrameUpgradeWarning=on
  COMM_OK : Outport
  COMM_DONE : Outport  Port=2
  wires:
  Gain4/1 -> Abs/1
  DirectionCompensation2/1(Out1) -> Gain4/1
  Sum4/1 -> DirectionCompensation2/1(In1)  "Delta_rad"
  Gain3/1 -> Sum4/2
  Constant7/1 -> Gain3/1
  Constant3/1 -> Switch/3
  Sum5/1 -> Switch/1
  Unit Delay1/1 -> Sum5/1
  Constant4/1 -> Sum5/2
  Logical Operator1/1 -> Unit Delay2/1, COMM_DONE/1
  Compare To Constant2/1 -> Logical Operator1/1
  Switch/1 -> Unit Delay1/1, Compare To Constant2/1
  Unit Delay2/1 -> Logical Operator1/2
  Sum3/1 -> Compare To Constant/1
  Compare To Constant/1 -> Scope/1, Logical Operator/1
  Abs/1 -> Compare To Constant1/1
  Product/1 -> Gain/1
  Compare To Constant1/1 -> Scope/2, Logical Operator/2
  Constant/1 -> Sum/2
  Logical Operator/1 -> Switch/2, COMM_OK/1
  Bus Selector2/1 -> Sum/1  "<x_m>"
  Bus Selector2/2 -> Sum1/1  "<y_m>"
  Constant1/1 -> Sum1/2
  X/1 -> Bus Selector2/1
  Sum1/1 -> Product1/1, Product1/2
  Gain/1 -> Sum3/1
  Sum/1 -> Product/1, Product/2
  Gain1/1 -> Sum3/2
  Bus Selector2/3 -> Sum4/1  "<tht_rad>"
  Product1/1 -> Gain1/1

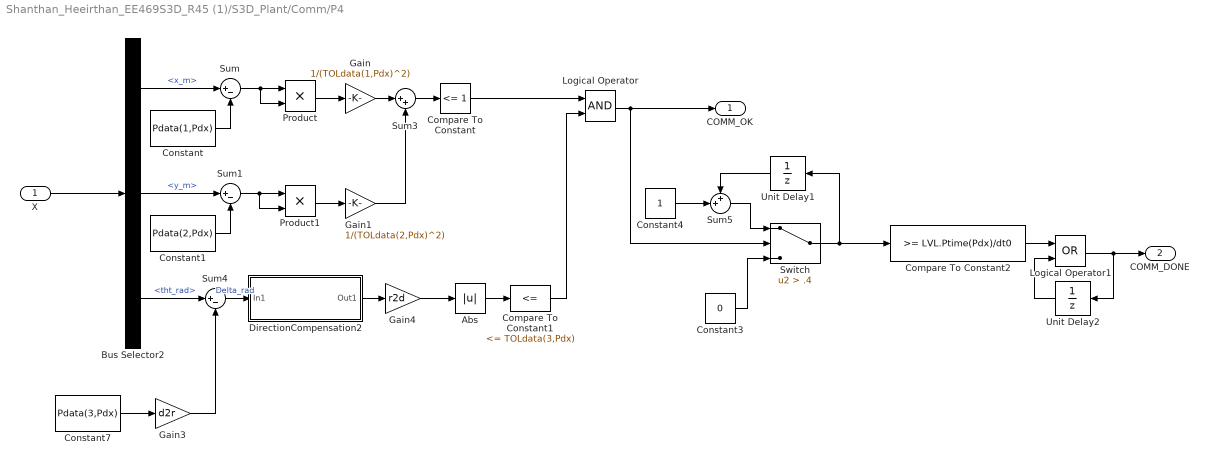
== system Shanthan_Heeirthan_EE469S3D_R45 (1)/S3D_Plant/Comm/P4 ==
  X : Inport
  Abs : Abs  SaturateOnIntegerOverflow=off
  Bus Selector2 : BusSelector  OutputSignals=x_m,y_m,tht_rad
  Compare To Constant : simulink/Logic and Bit Operations/Compare To Constant  relop=<=  const=1  OutDataTypeStr=boolean
  Compare To Constant1 : simulink/Logic and Bit Operations/Compare To Constant  relop=<=  const=TOLdata(3,Pdx)  OutDataTypeStr=boolean
  Compare To Constant2 : simulink/Logic and Bit Operations/Compare To Constant  relop=>=  const=LVL.Ptime(Pdx)/dt0  OutDataTypeStr=boolean
  Constant : Constant  Value=Pdata(1,Pdx)  SampleTime=dt0
  Constant1 : Constant  Value=Pdata(2,Pdx)  SampleTime=dt0
  Constant3 : Constant  Value=0  SampleTime=dt0
  Constant4 : Constant  SampleTime=dt0
  Constant7 : Constant  Value=Pdata(3,Pdx)  SampleTime=dt0
  DirectionCompensation2 : Subsystem
  Gain : Gain  Gain=1/(TOLdata(1,Pdx)^2)
  Gain1 : Gain  Gain=1/(TOLdata(2,Pdx)^2)
  Gain3 : Gain  Gain=d2r
  Gain4 : Gain  Gain=r2d
  Logical Operator : Logic  AllPortsSameDT=off  OutDataTypeStr=boolean
  Logical Operator1 : Logic  Operator=OR  AllPortsSameDT=off  OutDataTypeStr=boolean
  Product : Product
  Product1 : Product
  Sum : Sum  Inputs=|+-
  Sum1 : Sum  Inputs=|+-
  Sum3 : Sum  Inputs=|++
  Sum4 : Sum  Inputs=|+-
  Sum5 : Sum  Inputs=++|
  Switch : Switch  Criteria=u2 > Threshold  Threshold=.4  SaturateOnIntegerOverflow=off  InputSameDT=off
  Unit Delay1 : UnitDelay  SampleTime=dt0  HasFrameUpgradeWarning=on
  Unit Delay2 : UnitDelay  SampleTime=dt0  HasFrameUpgradeWarning=on
  COMM_OK : Outport
  COMM_DONE : Outport  Port=2
  wires:
  Gain4/1 -> Abs/1
  DirectionCompensation2/1(Out1) -> Gain4/1
  Sum4/1 -> DirectionCompensation2/1(In1)  "Delta_rad"
  Gain3/1 -> Sum4/2
  Constant7/1 -> Gain3/1
  Constant3/1 -> Switch/3
  Sum5/1 -> Switch/1
  Unit Delay1/1 -> Sum5/1
  Constant4/1 -> Sum5/2
  Logical Operator1/1 -> Unit Delay2/1, COMM_DONE/1
  Compare To Constant2/1 -> Logical Operator1/1
  Switch/1 -> Unit Delay1/1, Compare To Constant2/1
  Unit Delay2/1 -> Logical Operator1/2
  Sum3/1 -> Compare To Constant/1
  Compare To Constant/1 -> Logical Operator/1
  Abs/1 -> Compare To Constant1/1
  Product/1 -> Gain/1
  Compare To Constant1/1 -> Logical Operator/2
  Constant/1 -> Sum/2
  Logical Operator/1 -> Switch/2, COMM_OK/1
  Bus Selector2/1 -> Sum/1  "<x_m>"
  Bus Selector2/2 -> Sum1/1  "<y_m>"
  Constant1/1 -> Sum1/2
  X/1 -> Bus Selector2/1
  Sum1/1 -> Product1/1, Product1/2
  Gain/1 -> Sum3/1
  Sum/1 -> Product/1, Product/2
  Gain1/1 -> Sum3/2
  Bus Selector2/3 -> Sum4/1  "<tht_rad>"
  Product1/1 -> Gain1/1

== system Shanthan_Heeirthan_EE469S3D_R45 (1)/S3D_Plant/GetAccel/GetFxb ==
  U : Inport
  Bus Selector : BusSelector  OutputSignals=U1,U2,U3,U4
  Sum : Sum  Inputs=|++
  Sum1 : Sum  Inputs=|++
  Sum2 : Sum  Inputs=|+-
  Fxb : Outport
  wires:
  Bus Selector/3 -> Sum1/1  "<U3>"
  Sum2/1 -> Fxb/1  "Fxb_N"
  Bus Selector/1 -> Sum/1  "<U1>"
  Bus Selector/2 -> Sum/2  "<U2>"
  Sum1/1 -> Sum2/2
  Bus Selector/4 -> Sum1/2  "<U4>"
  Sum/1 -> Sum2/1
  U/1 -> Bus Selector/1

== system Shanthan_Heeirthan_EE469S3D_R45 (1)/S3D_Plant/GetAccel/GetFyb ==
  U : Inport
  Bus Selector : BusSelector  OutputSignals=U5,U8,U6,U7
  Sum3 : Sum  Inputs=|++
  Sum4 : Sum  Inputs=|++
  Sum5 : Sum  Inputs=|-+
  Fyb : Outport
  wires:
  U/1 -> Bus Selector/1
  Bus Selector/4 -> Sum4/2  "<U7>"
  Bus Selector/2 -> Sum3/2  "<U8>"
  Sum3/1 -> Sum5/1
  Sum4/1 -> Sum5/2
  Bus Selector/3 -> Sum4/1  "<U6>"
  Bus Selector/1 -> Sum3/1  "<U5>"
  Sum5/1 -> Fyb/1  "Fyb_N"

== system Shanthan_Heeirthan_EE469S3D_R45 (1)/S3D_Plant/GetAccel/GetMz ==
  U : Inport
  MP : Inport  Port=2
  Bus Selector : BusSelector  OutputSignals=U1,U2,U3,U4,U5,U6,U7,U8  OutputAsBus=on
  Bus Selector3 : BusSelector  OutputSignals=Ycg_m
  Bus Selector4 : BusSelector  OutputSignals=Xcg_m
  Bus to Vector : BusToVector
  Constant1 : Constant  Value=[-1 1 -1 1]  SampleTime=dt0
  Constant2 : Constant  Value=[1 1 -1 -1]  SampleTime=dt0
  Constant3 : Constant  Value=[3 -3 3 -3]  SampleTime=dt0
  Constant4 : Constant  Value=[1 -1 -1 1]  SampleTime=dt0
  Dot Product3 : DotProduct  OutDataTypeStr=Inherit: Inherit via internal rule
  Mux : Mux  Inputs=2
  Product2 : Product
  Product3 : Product
  Sum7 : Sum  Inputs=|++
  Sum8 : Sum  Inputs=|++
  Mzb : Outport
  wires:
  Dot Product3/1 -> Mzb/1  "Mzb_Nm"
  Mux/1 -> Dot Product3/2
  Bus to Vector/1 -> Dot Product3/1
  Bus Selector/1 -> Bus to Vector/1
  Sum8/1 -> Mux/2
  Sum7/1 -> Mux/1
  Product3/1 -> Sum8/2
  Constant3/1 -> Sum8/1
  Bus Selector4/1 -> Product3/2  "<Xcg_m>"
  Constant4/1 -> Product3/1
  MP/1 -> Bus Selector3/1, Bus Selector4/1
  Product2/1 -> Sum7/2
  Constant1/1 -> Sum7/1
  Bus Selector3/1 -> Product2/2  "<Ycg_m>"
  Constant2/1 -> Product2/1
  U/1 -> Bus Selector/1

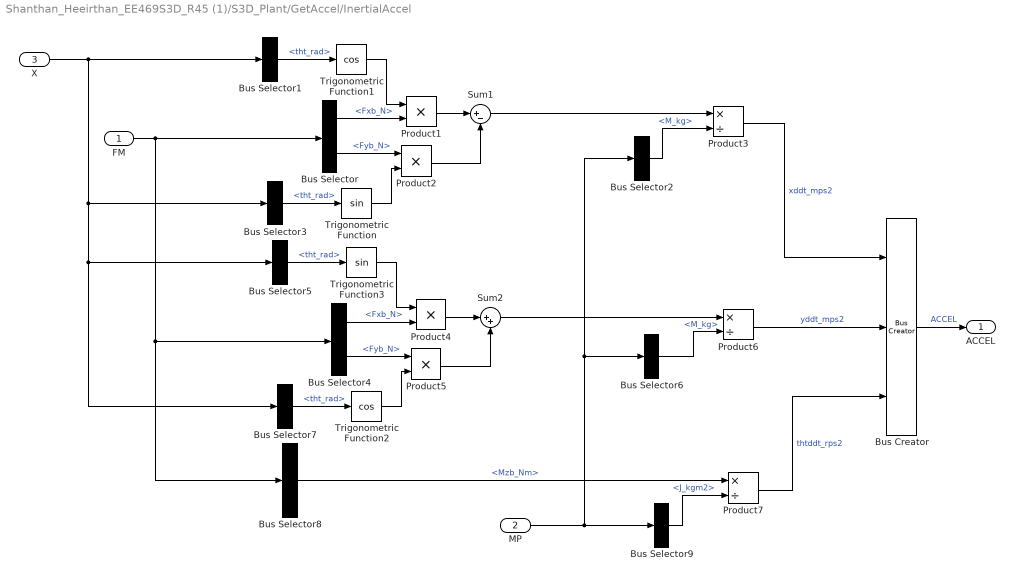
== system Shanthan_Heeirthan_EE469S3D_R45 (1)/S3D_Plant/GetAccel/InertialAccel ==
  FM : Inport
  MP : Inport  Port=2
  X : Inport  Port=3
  Bus Creator : BusCreator  Inputs=3
  Bus Selector : BusSelector  OutputSignals=Fxb_N,Fyb_N
  Bus Selector{1,3,5,7} (4 alike) : BusSelector  OutputSignals=tht_rad
  Bus Selector2 : BusSelector  OutputSignals=M_kg
  Bus Selector4 : BusSelector  OutputSignals=Fxb_N,Fyb_N
  Bus Selector6 : BusSelector  OutputSignals=M_kg
  Bus Selector8 : BusSelector  OutputSignals=Mzb_Nm
  Bus Selector9 : BusSelector  OutputSignals=J_kgm2
  Product{1..2,4..5} (4 alike) : Product
  Product3 : Product  Inputs=*/
  Product6 : Product  Inputs=*/
  Product7 : Product  Inputs=*/
  Sum1 : Sum  Inputs=|+-
  Sum2 : Sum  Inputs=|++
  Trigonometric Function : Trigonometry
  Trigonometric Function1 : Trigonometry  Operator=cos
  Trigonometric Function2 : Trigonometry  Operator=cos
  Trigonometric Function3 : Trigonometry
  ACCEL : Outport
  wires:
  Bus Creator/1 -> ACCEL/1  "ACCEL"
  Product7/1 -> Bus Creator/3  "thtddt_rps2"
  Product3/1 -> Bus Creator/1  "xddt_mps2"
  Product6/1 -> Bus Creator/2  "yddt_mps2"
  Bus Selector6/1 -> Product6/2  "<M_kg>"
  FM/1 -> Bus Selector/1, Bus Selector4/1, Bus Selector8/1
  Bus Selector9/1 -> Product7/2  "<J_kgm2>"
  Bus Selector8/1 -> Product7/1  "<Mzb_Nm>"
  Bus Selector7/1 -> Trigonometric Function2/1  "<tht_rad>"
  Sum2/1 -> Product6/1
  Bus Selector5/1 -> Trigonometric Function3/1  "<tht_rad>"
  Product4/1 -> Sum2/1
  Bus Selector4/1 -> Product4/2  "<Fxb_N>"
  Bus Selector4/2 -> Product5/1  "<Fyb_N>"
  Trigonometric Function2/1 -> Product5/2
  X/1 -> Bus Selector3/1, Bus Selector5/1, Bus Selector7/1, Bus Selector1/1
  Product5/1 -> Sum2/2
  Trigonometric Function3/1 -> Product4/1
  Trigonometric Function1/1 -> Product1/1
  Product2/1 -> Sum1/2
  Trigonometric Function/1 -> Product2/2
  Bus Selector/2 -> Product2/1  "<Fyb_N>"
  Bus Selector/1 -> Product1/2  "<Fxb_N>"
  MP/1 -> Bus Selector9/1, Bus Selector6/1, Bus Selector2/1
  Product1/1 -> Sum1/1
  Bus Selector1/1 -> Trigonometric Function1/1  "<tht_rad>"
  Bus Selector2/1 -> Product3/2  "<M_kg>"
  Sum1/1 -> Product3/1
  Bus Selector3/1 -> Trigonometric Function/1  "<tht_rad>"

== system Shanthan_Heeirthan_EE469S3D_R45 (1)/S3D_Plant/Integrate/ABM_INT1 ==
  DX : Inport
  Gain : Gain  Gain=23
  Gain1 : Gain  Gain=16
  Gain2 : Gain  Gain=5
  Product : Product  RndMeth=Zero
  Sum : Sum  Inputs=+-+
  Sum2 : Sum  Inputs=++|
  Unit Delay : UnitDelay  SampleTime=dt0  HasFrameUpgradeWarning=on
  Unit Delay1 : UnitDelay  SampleTime=dt0  HasFrameUpgradeWarning=on
  Unit Delay2 : UnitDelay  SampleTime=dt0  HasFrameUpgradeWarning=on
  dt/12 : Constant  Value=dt0/12  SampleTime=dt0
  X : Outport
  wires:
  Gain/1 -> Sum/1
  Gain2/1 -> Sum/3
  Gain1/1 -> Sum/2
  Sum/1 -> Product/2
  DX/1 -> Gain/1, Unit Delay1/1
  Unit Delay/1 -> X/1, Sum2/1  "X"
  Product/1 -> Sum2/2
  Unit Delay1/1 -> Gain1/1, Unit Delay2/1
  Unit Delay2/1 -> Gain2/1
  dt/12/1 -> Product/1
  Sum2/1 -> Unit Delay/1

== system Shanthan_Heeirthan_EE469S3D_R45 (1)/S3D_Plant/Integrate/CentroidData ==
  MP : Inport
  XCG : Inport  Port=2
  Bus Creator : BusCreator  Inputs=9
  Bus Selector4 : BusSelector  OutputSignals=tht_rad,thtdt_rps,thtddt_rps2
  FindCentroid : Subsystem
  FindCentroidAccel : Subsystem
  FindCentroidRates : Subsystem
  XCentroid : Outport
  wires:
  Bus Selector4/3 -> Bus Creator/9  "<thtddt_rps2>"
  Bus Selector4/2 -> Bus Creator/8  "<thtdt_rps>"
  Bus Selector4/1 -> Bus Creator/7  "<tht_rad>"
  FindCentroidAccel/1(Xddtcentroid) -> Bus Creator/5
  FindCentroidAccel/2(Yddtcentroid) -> Bus Creator/6
  FindCentroidRates/1(Xdtcentroid) -> Bus Creator/3
  FindCentroidRates/2(Ydtcentroid) -> Bus Creator/4
  FindCentroid/2(Ycentroid) -> Bus Creator/2
  FindCentroid/1(Xcentroid) -> Bus Creator/1
  XCG/1 -> FindCentroid/2(XCG), FindCentroidRates/2(XCG), FindCentroidAccel/2(XCG), Bus Selector4/1
  MP/1 -> FindCentroid/1(MP), FindCentroidRates/1(MP), FindCentroidAccel/1(MP)
  Bus Creator/1 -> XCentroid/1  "XCentroid"

== system Shanthan_Heeirthan_EE469S3D_R45 (1)/S3D_Plant/MassProperties/GetCGnJ ==
  MfuelVector : Inport
  M_kg : Inport  Port=2
  Constant1 : Constant  Value=[L13 L24 L13 L24].^2  SampleTime=dt0
  Constant2 : Constant  Value=[-3 -2 3 2]  SampleTime=dt0
  Constant3 : Constant  Value=[1 -1.5 -1 1.5]  SampleTime=dt0
  Constant4 : Constant  Value=[17 8 17 8]./12  SampleTime=dt0
  Constant5 : Constant  Value=Jbase+JC0  SampleTime=dt0
  Dot Product{,1..3} (4 alike) : DotProduct  OutDataTypeStr=Inherit: Inherit via internal rule
  Subsystem : Subsystem
  Sum1 : Sum  Inputs=+++
  Sum2 : Sum  Inputs=|++
  Xcg : Outport
  Ycg : Outport  Port=2
  J : Outport  Port=3
  wires:
  MfuelVector/1 -> Dot Product1/2, Dot Product/2, Dot Product3/2, Dot Product2/2
  Sum2/1 -> J/1  "J_kgm2"
  Subsystem/1(Jpat) -> Sum2/2
  Sum1/1 -> Sum2/1
  Constant5/1 -> Sum1/1
  Dot Product3/1 -> Sum1/2
  Dot Product2/1 -> Sum1/3
  Constant1/1 -> Dot Product2/1
  Constant4/1 -> Dot Product3/1
  Subsystem/3(Ycg) -> Ycg/1
  Subsystem/2(Xcg) -> Xcg/1
  M_kg/1 -> Subsystem/3(M_kg)
  Dot Product1/1 -> Subsystem/2(Ymom)  "Ymom"
  Dot Product/1 -> Subsystem/1(Xmom)  "Xmom"
  Constant3/1 -> Dot Product1/1
  Constant2/1 -> Dot Product/1

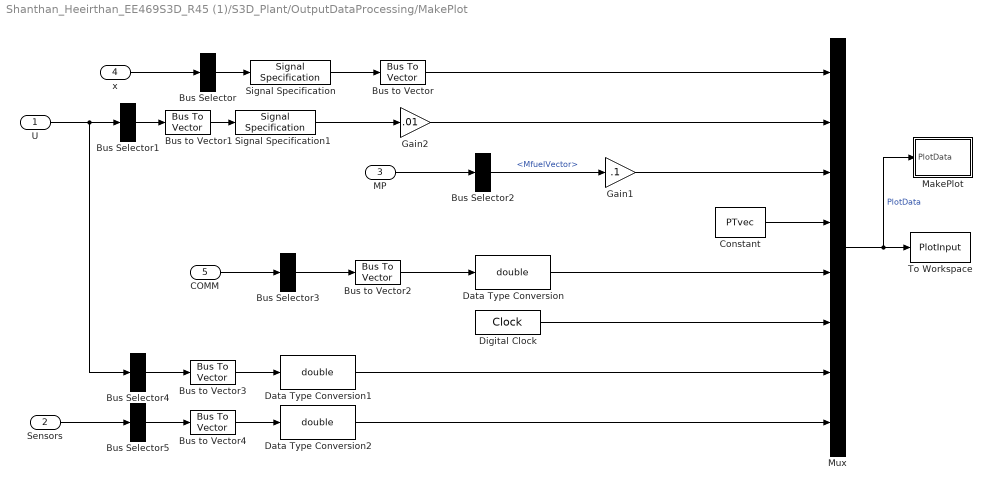
== system Shanthan_Heeirthan_EE469S3D_R45 (1)/S3D_Plant/OutputDataProcessing/MakePlot ==
  U : Inport
  Sensors : Inport  Port=2
  MP : Inport  Port=3
  x : Inport  Port=4
  COMM : Inport  Port=5
  Bus Selector : BusSelector  OutputSignals=x_m,y_m,tht_rad  OutputAsBus=on
  Bus Selector1 : BusSelector  OutputSignals=U1,U2,U3,U4,U5,U6,U7,U8  OutputAsBus=on
  Bus Selector2 : BusSelector  OutputSignals=MfuelVector
  Bus Selector3 : BusSelector  OutputSignals=P1OK,P1Done,P2OK,P2Done,P3OK,P3Done,P4OK,P4Done  OutputAsBus=on
  Bus Selector4 : BusSelector  OutputSignals=U1fail,U2fail,U3fail,U4fail,U5fail,U6fail,U7fail,U8fail  OutputAsBus=on
  Bus Selector5 : BusSelector  OutputSignals=S1fail,S2fail,S3fail,S4fail,S5fail,S6fail,S7fail,S8fail,S9fail  OutputAsBus=on
  Bus to Vector{,1..4} (5 alike) : BusToVector
  Constant : Constant  Value=PTvec  SampleTime=dt0
  Data Type Conversion : DataTypeConversion  OutDataTypeStr=double  SaturateOnIntegerOverflow=off  RndMeth=Floor
  Data Type Conversion1 : DataTypeConversion  OutDataTypeStr=double  SaturateOnIntegerOverflow=off  RndMeth=Floor
  Data Type Conversion2 : DataTypeConversion  OutDataTypeStr=double  SaturateOnIntegerOverflow=off  RndMeth=Floor
  Digital Clock : DigitalClock  SampleTime=dt0
  Gain1 : Gain  Gain=.1
  Gain2 : Gain  Gain=.01
  MakePlot : Subsystem
  Mux : Mux  Inputs=8
  Signal Specification : SignalSpecification  Dimensions=[3]
  Signal Specification1 : SignalSpecification  Dimensions=[8]
  To Workspace : ToWorkspace  VariableName=PlotInput  SampleTime=dt0
      settings: MaxDataPoints=1
  wires:
  Data Type Conversion/1 -> Mux/5
  Bus to Vector2/1 -> Data Type Conversion/1
  Bus Selector3/1 -> Bus to Vector2/1
  COMM/1 -> Bus Selector3/1
  Signal Specification1/1 -> Gain2/1
  Constant/1 -> Mux/4
  Gain1/1 -> Mux/3
  Signal Specification/1 -> Bus to Vector/1
  Bus Selector2/1 -> Gain1/1  "<MfuelVector>"
  MP/1 -> Bus Selector2/1
  Bus to Vector1/1 -> Signal Specification1/1
  Bus Selector1/1 -> Bus to Vector1/1
  U/1 -> Bus Selector4/1, Bus Selector1/1
  Bus to Vector/1 -> Mux/1
  Bus Selector/1 -> Signal Specification/1
  Gain2/1 -> Mux/2
  x/1 -> Bus Selector/1
  Mux/1 -> MakePlot/1(PlotData), To Workspace/1  "PlotData"
  Digital Clock/1 -> Mux/6
  Bus Selector4/1 -> Bus to Vector3/1
  Bus to Vector3/1 -> Data Type Conversion1/1
  Data Type Conversion1/1 -> Mux/7
  Bus to Vector4/1 -> Data Type Conversion2/1
  Bus Selector5/1 -> Bus to Vector4/1
  Sensors/1 -> Bus Selector5/1
  Data Type Conversion2/1 -> Mux/8
